simulink model "CariIMP"  (R2023b)
settings: Solver=VariableStepAuto  StartTime=0.0  StopTime=30  RelTol=1e-3
values from neighbouring files (symbols this model uses):
  A = [         Ap           Bp*Ca ... (first row only)    [FindIMP.m]    (also in cobacobaIMP.m)
  B = [zeros(p_size,a_size) ... (first row only)    [FindIMP.m]    (also in cobacobaIMP.m)
  C = [Cp zeros(2,a_size)]    [FindIMP.m]    (also in cobacobaIMP.m)
undefined symbols (not defined in the file or in its folder): K_base, K_opt, V, xr0
libraries: simulink x1
settings Model: Creator=izmah  LastModifiedBy=izmah

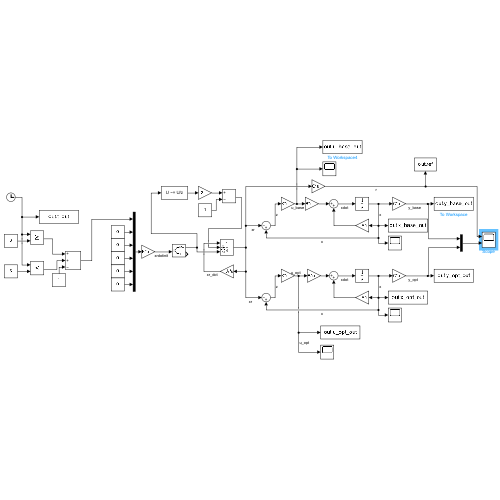
[thumbnail: Simulink's stored preview of the top-level diagram]
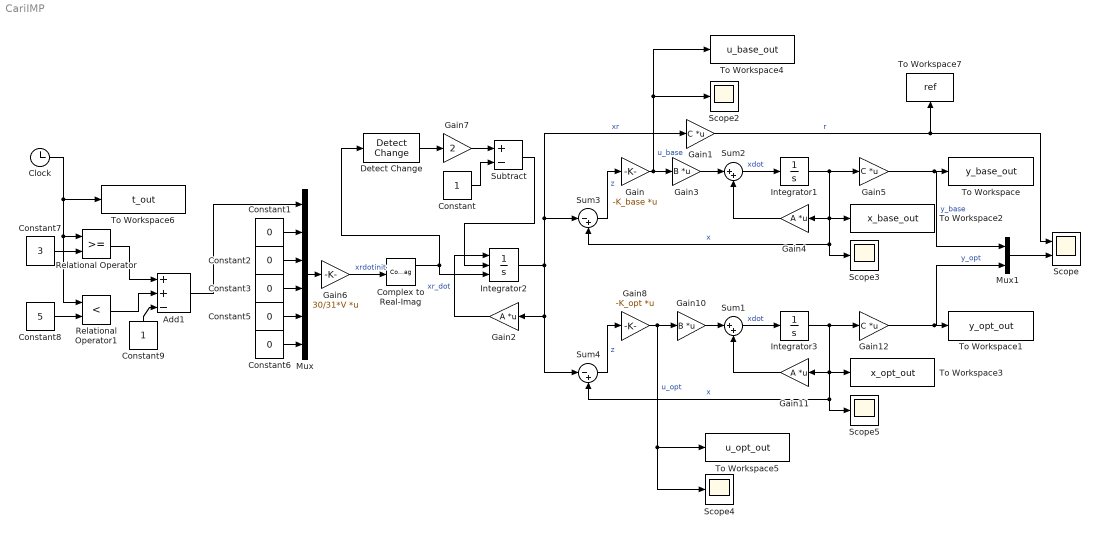
== system CariIMP ==
  Add1 : Sum  Inputs=++-
  Clock : Clock
  Complex to Real-Imag : ComplexToRealImag
  Constant : Constant
  Constant{1..3,5..6} (5 alike) : Constant  Value=0
  Constant7 : Constant  Value=3
  Constant8 : Constant  Value=5
  Constant9 : Constant
  Detect Change : simulink/Logic and Bit Operations/Detect Change  vinit=0  OutDataTypeStr=boolean
  Gain : Gain  Gain=-K_base  Multiplication=Matrix(K*u)
  Gain1 : Gain  Gain=C  Multiplication=Matrix(K*u)
  Gain10 : Gain  Gain=B  Multiplication=Matrix(K*u)
  Gain11 : Gain  Gain=A  Multiplication=Matrix(K*u)
  Gain12 : Gain  Gain=C  Multiplication=Matrix(K*u)
  Gain2 : Gain  Gain=A  Multiplication=Matrix(K*u)
  Gain3 : Gain  Gain=B  Multiplication=Matrix(K*u)
  Gain4 : Gain  Gain=A  Multiplication=Matrix(K*u)
  Gain5 : Gain  Gain=C  Multiplication=Matrix(K*u)
  Gain6 : Gain  Gain=30/31*V  Multiplication=Matrix(K*u)
  Gain7 : Gain  Gain=2
  Gain8 : Gain  Gain=-K_opt  Multiplication=Matrix(K*u)
  Integrator1 : Integrator
  Integrator2 : Integrator  ExternalReset=either  InitialConditionSource=external  InitialCondition=xr0  ZeroCross=off
  Integrator3 : Integrator
  Mux : Mux  Inputs=6
  Mux1 : Mux  Inputs=2
  Relational Operator : RelationalOperator  OutDataTypeStr=boolean  RndMeth=Simplest  InputSameDT=off
  Relational Operator1 : RelationalOperator  Operator=<  OutDataTypeStr=boolean  RndMeth=Simplest  InputSameDT=off
  Scope : Scope  NumInputPorts=2
  Scope{2..5} (4 alike) : Scope
  Subtract : Sum  Inputs=+-
  Sum1 : Sum  Inputs=|++
  Sum2 : Sum  Inputs=|++
  Sum3 : Sum  Inputs=|-+
  Sum4 : Sum  Inputs=|-+
  To Workspace : ToWorkspace  VariableName=y_base_out  SampleTime=-1
  To Workspace1 : ToWorkspace  VariableName=y_opt_out  SampleTime=-1
  To Workspace2 : ToWorkspace  VariableName=x_base_out  SampleTime=-1
  To Workspace3 : ToWorkspace  VariableName=x_opt_out  SampleTime=-1
  To Workspace4 : ToWorkspace  VariableName=u_base_out  SampleTime=-1
  To Workspace5 : ToWorkspace  VariableName=u_opt_out  SampleTime=-1
  To Workspace6 : ToWorkspace  VariableName=t_out  SampleTime=-1
  To Workspace7 : ToWorkspace  VariableName=ref  SampleTime=-1
  wires:
  Sum2/1 -> Integrator1/1  "xdot"
  Gain3/1 -> Sum2/1
  Gain4/1 -> Sum2/2
  Integrator1/1 -> Gain5/1, Scope3/1, Sum3/2, To Workspace2/1, Gain4/1  "x"
  Gain2/1 -> Integrator2/1  "xr_dot"
  Integrator2/1 -> Sum4/1, Gain2/1, Sum3/1, Gain1/1  "xr"
  Sum3/1 -> Gain/1  "z"
  Constant1/1 -> Mux/2
  Constant2/1 -> Mux/3
  Constant3/1 -> Mux/4
  Constant5/1 -> Mux/5
  Constant6/1 -> Mux/6
  Mux/1 -> Gain6/1
  Gain5/1 -> To Workspace/1, Mux1/1  "y_base"
  Gain1/1 -> Scope/1, To Workspace7/1  "r"
  Complex to Real-Imag/1 -> Integrator2/3, Detect Change/1
  Gain6/1 -> Complex to Real-Imag/1  "xrdotinit"
  Constant/1 -> Subtract/2
  Detect Change/1 -> Gain7/1
  Subtract/1 -> Integrator2/2
  Gain7/1 -> Subtract/1
  Clock/1 -> Relational Operator/1, Relational Operator1/1, To Workspace6/1
  Constant8/1 -> Relational Operator1/2
  Constant7/1 -> Relational Operator/2
  Relational Operator1/1 -> Add1/2
  Constant9/1 -> Add1/3
  Relational Operator/1 -> Add1/1
  Add1/1 -> Mux/1
  Gain11/1 -> Sum1/2
  Integrator3/1 -> Gain12/1, Scope5/1, Sum4/2, To Workspace3/1, Gain11/1  "x"
  Gain12/1 -> To Workspace1/1, Mux1/2  "y_opt"
  Sum1/1 -> Integrator3/1  "xdot"
  Gain10/1 -> Sum1/1
  Sum4/1 -> Gain8/1  "z"
  Mux1/1 -> Scope/2
  Gain8/1 -> Scope4/1, To Workspace5/1, Gain10/1  "u_opt"
  Gain/1 -> Gain3/1, To Workspace4/1, Scope2/1  "u_base"
